simulink model "CMOS_Kernel_Memory_Sync"  (R2023b)
settings: Solver=VariableStepAuto  StartTime=0.0  StopTime=30000000  RelTol=1e-3
values from neighbouring files (symbols this model uses):
  AmountOfPixelsPerScanline = 400    [Kernel_Setup_Script.m]
  AmountOfRamBlocksScanlines = 5    [Kernel_Setup_Script.m]
  AmountOfRamBlocksScanlinesOffset = AmountOfRamBlocksScanlines - 1    (= 4)    [Kernel_Setup_Script.m]
  AmountOfScanlinePixels = 73700    [Kernel_Setup_Script.m]
  AmountOfScanlinePixelsOffset = AmountOfScanlinePixels - 1    (= 73699)    [Kernel_Setup_Script.m]
  AmountOfScanlines = 1100    [Kernel_Setup_Script.m]
  AmountOfScanlinesOffset = AmountOfScanlines - 1    (= 1099)    [Kernel_Setup_Script.m]
  AOPPK_Off = AmountOfPixelsPerScanline - 1    (= 399)    [Kernel_Setup_Script.m]
  AOPPS_Off = AmountOfPixelsPerScanline - 1    (= 399)    [Kernel_Setup_Script.m]
  FramePackOff_0 = FramePackOff_0 - ScanlineFifoCheck    [Kernel_Setup_Script.m]
  FramePackOff_1 = FramePackOff_1 - ScanlineFifoCheck    [Kernel_Setup_Script.m]
  FramePackOff_2 = FramePackOff_2 - ScanlineFifoCheck    [Kernel_Setup_Script.m]
  FramePackOff_3 = FramePackOff_3 - ScanlineFifoCheck    [Kernel_Setup_Script.m]
  FramePackOff_4 = FramePackOff_4 - ScanlineFifoCheck    [Kernel_Setup_Script.m]
  FramePackOff_5 = FramePackOff_5 - ScanlineFifoCheck    [Kernel_Setup_Script.m]
  KernelPackOff_0 = KernelPackOff_0 - KernelBitsPerRow    [Kernel_Setup_Script.m]
  KernelPackOff_1 = KernelPackOff_1 - KernelBitsPerRow    [Kernel_Setup_Script.m]
  KernelPackOff_2 = KernelPackOff_2 - KernelBitsPerRow    [Kernel_Setup_Script.m]
  KernelPackOff_3 = KernelPackOff_3 - KernelBitsPerRow    [Kernel_Setup_Script.m]
  Slice59DownTo48Top = (MsbOffset - (ScanlinePixelBitSizeController*1))    (= 59)    [Kernel_Setup_Script.m]
  Slice71DownTo60Top = (MsbOffset - (ScanlinePixelBitSizeController*0))    (= 71)    [Kernel_Setup_Script.m]
  TotalSectionsForFrames = AmountOfScanlines/AmountOfRamBlocksScanlines    (= 220)    [Kernel_Setup_Script.m]
  UltraRamRows = AmountOfPixelsPerScanline/ScanlineFifoCheck    [Kernel_Setup_Script.m]
  UltraRamRowsCeil = ceil(AmountOfPixelsPerScanline/ScanlineFifoCheck)    [Kernel_Setup_Script.m]
  UltraRamRowsKernel = AmountOfPixelsPerScanline/KernelBitsPerRow    (= 100)    [Kernel_Setup_Script.m]
  UltraRamRowsKernelCeil = ceil(AmountOfPixelsPerScanline/KernelBitsPerRow)    [Kernel_Setup_Script.m]
  UltraRamRowsMemorySectionOffset = UltraRamRowsCeil*AmountOfRamBlocksScanlines    [Kernel_Setup_Script.m]
  UltraRamRowsOffset = UltraRamRowsCeil - 1    [Kernel_Setup_Script.m]
undefined symbols (not defined in the file or in its folder): c, Down, sfvc784, Up, xck26
libraries: hdlBasic x4512, vmcUtilities x1
(part 14 of 39)

== system CMOS_Kernel_Memory_Sync/Memory Handler/Data Slicer/Frame RAM Slicer/72 Bit Unpacker RAM 4 ==
  Data In : Inport
  Enable : Inport  Port=2
  Read Enable : Inport  Port=3
  Last Point : Inport  Port=4
  72bit Frame FIFO 0 : hdlBasic/FIFO  mem_type=Block RAM  performance_options=Standard_FIFO  embedded_registers=off  depth=16  use_asym_data_widths=off  asym_read_width=32  percent_nbits=1  rst=off  rst_latency=2  en=off  use_dcount=off  use_percent_full_port=off  use_almost_empty=off  almost_empty_thresh=2  use_almost_full=off  use_rd_rst_busy=off  use_wr_rst_busy=off  almost_full_thresh=14  almost_empty_offset=[]  almost_full_offset=[]  explicit_period=off  period=[]  store_only_valid=[]  init_zero=[]  simulation_type=fast_sim  XmcBlockStatus=1  maskContainerNames=tabcontainer1  block_type=fifo  block_config=sysgen:FIFO_config  block_width=538  block_height=997
      settings: infoedit=[]
  72bit Frame FIFO 1 : hdlBasic/FIFO  mem_type=Block RAM  performance_options=Standard_FIFO  embedded_registers=off  depth=16  use_asym_data_widths=off  asym_read_width=32  percent_nbits=1  rst=off  rst_latency=2  en=off  use_dcount=off  use_percent_full_port=off  use_almost_empty=off  almost_empty_thresh=2  use_almost_full=off  use_rd_rst_busy=off  use_wr_rst_busy=off  almost_full_thresh=14  almost_empty_offset=[]  almost_full_offset=[]  explicit_period=off  period=[]  store_only_valid=[]  init_zero=[]  simulation_type=fast_sim  XmcBlockStatus=1  maskContainerNames=tabcontainer1  block_type=fifo  block_config=sysgen:FIFO_config  block_width=538  block_height=997
      settings: infoedit=[]
  Bypass Delay : hdlBasic/Delay  rst=off  en=off  latency=1  reg_retiming=off  XmcBlockStatus=1  maskContainerNames=group1  block_type=delay  block_config=sysgen:Delay_config
  Bypass Delay1 : hdlBasic/Delay  rst=off  en=off  latency=1  reg_retiming=off  XmcBlockStatus=1  maskContainerNames=group1  block_type=delay  block_config=sysgen:Delay_config
  Bypass Delay2 : hdlBasic/Delay  rst=off  en=off  latency=1  reg_retiming=off  XmcBlockStatus=1  maskContainerNames=group1  block_type=delay  block_config=sysgen:Delay_config
  Data Delay : hdlBasic/Delay  rst=off  en=off  latency=1  reg_retiming=off  XmcBlockStatus=1  maskContainerNames=group1  block_type=delay  block_config=sysgen:Delay_config
  Data Enable Check : hdlBasic/Delay  rst=off  en=off  latency=1  reg_retiming=off  XmcBlockStatus=1  maskContainerNames=group1  block_type=delay  block_config=sysgen:Delay_config
  Data MUX Delay : hdlBasic/Delay  rst=off  en=off  latency=1  reg_retiming=off  XmcBlockStatus=1  maskContainerNames=group1  block_type=delay  block_config=sysgen:Delay_config
  Enable Delay : hdlBasic/Delay  rst=off  en=off  latency=1  reg_retiming=off  XmcBlockStatus=1  maskContainerNames=group1  block_type=delay  block_config=sysgen:Delay_config
  FIFO 0 : hdlBasic/Constant  const=0  gui_display_data_type=Fixed-point  arith_type=Unsigned  n_bits=1  bin_pt=0  preci_type=Single  exp_width=8  frac_width=24  explicit_period=off  period=1  XmcBlockStatus=1  maskContainerNames=tabcontainer1  block_type=constant  block_config=sysgen:Constant_config
  FIFO 1 : hdlBasic/Constant  const=1  gui_display_data_type=Fixed-point  arith_type=Unsigned  n_bits=1  bin_pt=0  preci_type=Single  exp_width=8  frac_width=24  explicit_period=off  period=1  XmcBlockStatus=1  maskContainerNames=tabcontainer1  block_type=constant  block_config=sysgen:Constant_config
  Last Point Delay 1 : hdlBasic/Delay  rst=off  en=off  latency=1  reg_retiming=off  XmcBlockStatus=1  maskContainerNames=group1  block_type=delay  block_config=sysgen:Delay_config
  Last Value Bypass FIFO 0 : hdlBasic/Logical  logical_function=OR  inputs=2  en=off  latency=1  precision=Full  arith_type=Unsigned  n_bits=16  bin_pt=0  align_bp=on  overflow=[]  quantization=[]  XmcBlockStatus=1  maskContainerNames=tabcontainer1  block_type=logical  block_config=sysgen:Logical_config
  Last Value Bypass FIFO 1 : hdlBasic/Logical  logical_function=OR  inputs=2  en=off  latency=1  precision=Full  arith_type=Unsigned  n_bits=16  bin_pt=0  align_bp=on  overflow=[]  quantization=[]  XmcBlockStatus=1  maskContainerNames=tabcontainer1  block_type=logical  block_config=sysgen:Logical_config
  Last Value Delay : hdlBasic/Delay  rst=off  en=off  latency=1  reg_retiming=off  XmcBlockStatus=1  maskContainerNames=group1  block_type=delay  block_config=sysgen:Delay_config
  Logical : hdlBasic/Logical  logical_function=NOR  inputs=2  en=off  latency=1  precision=Full  arith_type=Unsigned  n_bits=16  bin_pt=0  align_bp=on  overflow=[]  quantization=[]  XmcBlockStatus=1  maskContainerNames=tabcontainer1  block_type=logical  block_config=sysgen:Logical_config
  Store in FIFO 0 : hdlBasic/Relational  mode=a=b  op_type=Bool  en=off  latency=1  XmcBlockStatus=1  maskContainerNames=tabcontainer1  block_type=relational  block_config=sysgen:Relational_config
  Store in FIFO 1 : hdlBasic/Relational  mode=a=b  op_type=Bool  en=off  latency=1  XmcBlockStatus=1  maskContainerNames=tabcontainer1  block_type=relational  block_config=sysgen:Relational_config
  Sync Frame Counter : hdlBasic/Counter  cnt_type=Count limited  cnt_to=1  operation=Up  start_count=0  cnt_by_val=1  arith_type=Unsigned  n_bits=1  bin_pt=0  load_pin=off  rst=on  en=on  explicit_period=Explicit  period=1  use_behavioral_HDL=off  implementation=Fabric  XmcBlockStatus=1  maskContainerNames=group1  block_type=counter  block_config=sysgen:Counter_config  block_width=531  block_height=1023
  Unpack 72 Bit FIFO 0 : Subsystem
      settings: RTWMemSecFuncInitTerm=Inherit fRAM model  RTWMemSecFuncExecute=Inherit fRAM model  RTWMemSecDataConstants=Inherit fRAM model  RTWMemSecDataInternal=Inherit fRAM model  RTWMemSecDataParameters=Inherit fRAM model
  Unpack 72 Bit FIFO 1 : Subsystem
      settings: RTWMemSecFuncInitTerm=Inherit fRAM model  RTWMemSecFuncExecute=Inherit fRAM model  RTWMemSecDataConstants=Inherit fRAM model  RTWMemSecDataInternal=Inherit fRAM model  RTWMemSecDataParameters=Inherit fRAM model
  Valid : hdlBasic/Delay  rst=off  en=off  latency=1  reg_retiming=off  XmcBlockStatus=1  maskContainerNames=group1  block_type=delay  block_config=sysgen:Delay_config
  Write FIFO 0 MUX Delay : hdlBasic/Delay  rst=off  en=off  latency=1  reg_retiming=off  XmcBlockStatus=1  maskContainerNames=group1  block_type=delay  block_config=sysgen:Delay_config
  Write FIFO 1 MUX Delay : hdlBasic/Delay  rst=off  en=off  latency=1  reg_retiming=off  XmcBlockStatus=1  maskContainerNames=group1  block_type=delay  block_config=sysgen:Delay_config
  Write to FIFO 0 : hdlBasic/Logical  logical_function=AND  inputs=2  en=off  latency=1  precision=Full  arith_type=Unsigned  n_bits=16  bin_pt=0  align_bp=on  overflow=[]  quantization=[]  XmcBlockStatus=1  maskContainerNames=tabcontainer1  block_type=logical  block_config=sysgen:Logical_config
  Write to FIFO 1 : hdlBasic/Logical  logical_function=AND  inputs=2  en=off  latency=1  precision=Full  arith_type=Unsigned  n_bits=16  bin_pt=0  align_bp=on  overflow=[]  quantization=[]  XmcBlockStatus=1  maskContainerNames=tabcontainer1  block_type=logical  block_config=sysgen:Logical_config
  Zero FIFO Value : hdlBasic/Constant  const=0  gui_display_data_type=Fixed-point  arith_type=Unsigned  n_bits=72  bin_pt=0  preci_type=Single  exp_width=8  frac_width=24  explicit_period=off  period=1  XmcBlockStatus=1  maskContainerNames=tabcontainer1  block_type=constant  block_config=sysgen:Constant_config
  Zero Value : hdlBasic/Mux  inputs=2  en=off  latency=1  precision=Full  arith_type=Unsigned  n_bits=16  bin_pt=14  quantization=Truncate  overflow=Wrap  XmcBlockStatus=1  maskContainerNames=tabcontainer1  block_type=mux  block_config=sysgen:Mux_config
  71 Downto 60 FIFO 0 : Outport
  59 Downto 48 FIFO 0 : Outport  Port=2
  47 Downto 36 FIFO 0 : Outport  Port=3
  35 Downto 24 FIFO 0 : Outport  Port=4
  23 Downto 12 FIFO 0 : Outport  Port=5
  11 Downto 0 FIFO 0 : Outport  Port=6
  71 Downto 60 FIFO 1 : Outport  Port=7
  59 Downto 48 FIFO 1 : Outport  Port=8
  47 Downto 36 FIFO 1 : Outport  Port=9
  35 Downto 24 FIFO 1 : Outport  Port=10
  23 Downto 12 FIFO 1 : Outport  Port=11
  11 Downto 0 FIFO 1 : Outport  Port=12
  Valid Out : Outport  Port=13
  Wrote To a FIFO : Outport  Port=14
  wires:
  Sync Frame Counter/1 -> Store in FIFO 1/1, Store in FIFO 0/1
  Read Enable/1 -> 72bit Frame FIFO 0/3, 72bit Frame FIFO 1/3, Valid/1
  FIFO 1/1 -> Store in FIFO 1/2
  FIFO 0/1 -> Store in FIFO 0/2
  Write to FIFO 1/1 -> Write FIFO 1 MUX Delay/1
  Data Delay/1 -> Data Enable Check/1
  Data In/1 -> Data Delay/1
  Enable/1 -> Enable Delay/1, Sync Frame Counter/2
  72bit Frame FIFO 1/1 -> Unpack 72 Bit FIFO 1/1(72 Bit Input)
  72bit Frame FIFO 0/1 -> Unpack 72 Bit FIFO 0/1(72 Bit Input)
  Unpack 72 Bit FIFO 0/1(71 Downto 60) -> 71 Downto 60 FIFO 0/1
  Unpack 72 Bit FIFO 0/2(59 Downto 48) -> 59 Downto 48 FIFO 0/1
  Unpack 72 Bit FIFO 0/3(47 Downto 36) -> 47 Downto 36 FIFO 0/1
  Unpack 72 Bit FIFO 0/4(35 Downto 24) -> 35 Downto 24 FIFO 0/1
  Unpack 72 Bit FIFO 0/5(23 Downto 12) -> 23 Downto 12 FIFO 0/1
  Unpack 72 Bit FIFO 0/6(11 Downto 0) -> 11 Downto 0 FIFO 0/1
  Unpack 72 Bit FIFO 1/1(71 Downto 60) -> 71 Downto 60 FIFO 1/1
  Unpack 72 Bit FIFO 1/2(59 Downto 48) -> 59 Downto 48 FIFO 1/1
  Unpack 72 Bit FIFO 1/3(47 Downto 36) -> 47 Downto 36 FIFO 1/1
  Unpack 72 Bit FIFO 1/4(35 Downto 24) -> 35 Downto 24 FIFO 1/1
  Unpack 72 Bit FIFO 1/5(23 Downto 12) -> 23 Downto 12 FIFO 1/1
  Unpack 72 Bit FIFO 1/6(11 Downto 0) -> 11 Downto 0 FIFO 1/1
  Valid/1 -> Valid Out/1
  Write to FIFO 0/1 -> Write FIFO 0 MUX Delay/1
  Data Enable Check/1 -> Last Value Delay/1
  Enable Delay/1 -> Bypass Delay/1
  Last Point/1 -> Last Point Delay 1/1, Sync Frame Counter/1
  Last Value Delay/1 -> Data MUX Delay/1, Zero Value/2
  Last Value Bypass FIFO 0/1 -> Write to FIFO 0/1
  Store in FIFO 0/1 -> Last Value Bypass FIFO 0/1
  Last Value Bypass FIFO 1/1 -> Write to FIFO 1/2
  Store in FIFO 1/1 -> Last Value Bypass FIFO 1/1
  Last Point Delay 1/1 -> Last Value Bypass FIFO 1/2, Last Value Bypass FIFO 0/2, Bypass Delay1/1
  Bypass Delay/1 -> Write to FIFO 1/1, Write to FIFO 0/2
  Logical/1 -> Wrote To a FIFO/1
  72bit Frame FIFO 1/2 -> Logical/2
  72bit Frame FIFO 0/2 -> Logical/1
  Zero FIFO Value/1 -> Zero Value/3
  Zero Value/1 -> 72bit Frame FIFO 1/1
  Write FIFO 1 MUX Delay/1 -> 72bit Frame FIFO 1/2
  Write FIFO 0 MUX Delay/1 -> 72bit Frame FIFO 0/2
  Data MUX Delay/1 -> 72bit Frame FIFO 0/1
  Bypass Delay1/1 -> Bypass Delay2/1
  Bypass Delay2/1 -> Zero Value/1

== system CMOS_Kernel_Memory_Sync/Memory Handler/Data Slicer/Frame RAM Slicer/Data Point Tracker ==
  Data In RAM 0 : Inport
  Data In RAM 1 : Inport  Port=2
  Data In RAM 2 : Inport  Port=3
  Data In RAM 3 : Inport  Port=4
  Data In RAM 4 : Inport  Port=5
  Valid Enable In : Inport  Port=6
  Data In Delay 0 RAM {0..4} (5 alike) : hdlBasic/Delay  rst=off  en=off  latency=1  reg_retiming=off  XmcBlockStatus=1  maskContainerNames=group1  block_type=delay  block_config=sysgen:Delay_config
  Data In Delay 1 RAM {0..4} (5 alike) : hdlBasic/Delay  rst=off  en=off  latency=1  reg_retiming=off  XmcBlockStatus=1  maskContainerNames=group1  block_type=delay  block_config=sysgen:Delay_config
  Data Point Counter : hdlBasic/Counter  cnt_type=Count limited  cnt_to=UltraRamRowsCeil - 1  operation=Up  start_count=0  cnt_by_val=1  arith_type=Unsigned  n_bits=ceil(log2(UltraRamRowsCeil))  bin_pt=0  load_pin=off  rst=off  en=on  explicit_period=Explicit  period=1  use_behavioral_HDL=off  implementation=Fabric  XmcBlockStatus=1  maskContainerNames=group1  block_type=counter  block_config=sysgen:Counter_config  block_width=531  block_height=1023
  Last Data Point Value : hdlBasic/Constant  const=UltraRamRowsCeil - 1  gui_display_data_type=Fixed-point  arith_type=Unsigned  n_bits=ceil(log2(UltraRamRowsCeil))  bin_pt=0  preci_type=Single  exp_width=8  frac_width=24  explicit_period=off  period=1  XmcBlockStatus=1  maskContainerNames=tabcontainer1  block_type=constant  block_config=sysgen:Constant_config
  Last Point : hdlBasic/Relational  mode=a=b  op_type=Bool  en=off  latency=1  XmcBlockStatus=1  maskContainerNames=tabcontainer1  block_type=relational  block_config=sysgen:Relational_config
  Last Value enable : hdlBasic/Logical  logical_function=AND  inputs=2  en=off  latency=1  precision=Full  arith_type=Unsigned  n_bits=16  bin_pt=0  align_bp=on  overflow=[]  quantization=[]  XmcBlockStatus=1  maskContainerNames=tabcontainer1  block_type=logical  block_config=sysgen:Logical_config
  Valid Delay 0 : hdlBasic/Delay  rst=off  en=off  latency=1  reg_retiming=off  XmcBlockStatus=1  maskContainerNames=group1  block_type=delay  block_config=sysgen:Delay_config
  Valid Delay 1 : hdlBasic/Delay  rst=off  en=off  latency=1  reg_retiming=off  XmcBlockStatus=1  maskContainerNames=group1  block_type=delay  block_config=sysgen:Delay_config
  Data Out RAM 0 : Outport
  Data Out RAM 1 : Outport  Port=2
  Data Out RAM 2 : Outport  Port=3
  Data Out RAM 3 : Outport  Port=4
  Data Out RAM 4 : Outport  Port=5
  Valid Enable Out : Outport  Port=6
  Last Value Out : Outport  Port=7
  wires:
  Last Value enable/1 -> Last Value Out/1
  Data In Delay 0 RAM 1/1 -> Data In Delay 1 RAM 1/1
  Last Point/1 -> Last Value enable/2
  Data Point Counter/1 -> Last Point/1
  Valid Enable In/1 -> Valid Delay 0/1, Data Point Counter/1
  Data In Delay 0 RAM 2/1 -> Data In Delay 1 RAM 2/1
  Valid Delay 0/1 -> Last Value enable/1, Valid Delay 1/1
  Last Data Point Value/1 -> Last Point/2
  Data In Delay 0 RAM 4/1 -> Data In Delay 1 RAM 4/1
  Data In Delay 1 RAM 4/1 -> Data Out RAM 4/1
  Data In Delay 0 RAM 0/1 -> Data In Delay 1 RAM 0/1
  Data In Delay 0 RAM 3/1 -> Data In Delay 1 RAM 3/1
  Data In RAM 1/1 -> Data In Delay 0 RAM 1/1
  Data In Delay 1 RAM 0/1 -> Data Out RAM 0/1
  Data In RAM 3/1 -> Data In Delay 0 RAM 3/1
  Data In RAM 4/1 -> Data In Delay 0 RAM 4/1
  Data In RAM 2/1 -> Data In Delay 0 RAM 2/1
  Data In RAM 0/1 -> Data In Delay 0 RAM 0/1
  Data In Delay 1 RAM 2/1 -> Data Out RAM 2/1
  Data In Delay 1 RAM 3/1 -> Data Out RAM 3/1
  Data In Delay 1 RAM 1/1 -> Data Out RAM 1/1
  Valid Delay 1/1 -> Valid Enable Out/1

== system CMOS_Kernel_Memory_Sync/Memory Handler/Data Slicer/Kernel RAM Slicer/72 Bit Kernel Unpacker RAM 0 ==
  Data In : Inport
  Enable : Inport  Port=2
  Read Enable : Inport  Port=3
  Last Point : Inport  Port=4
  72bit Frame FIFO 0 : hdlBasic/FIFO  mem_type=Block RAM  performance_options=Standard_FIFO  embedded_registers=off  depth=16  use_asym_data_widths=off  asym_read_width=32  percent_nbits=1  rst=off  rst_latency=2  en=off  use_dcount=off  use_percent_full_port=off  use_almost_empty=off  almost_empty_thresh=2  use_almost_full=off  use_rd_rst_busy=off  use_wr_rst_busy=off  almost_full_thresh=14  almost_empty_offset=[]  almost_full_offset=[]  explicit_period=off  period=[]  store_only_valid=[]  init_zero=[]  simulation_type=fast_sim  XmcBlockStatus=1  maskContainerNames=tabcontainer1  block_type=fifo  block_config=sysgen:FIFO_config  block_width=538  block_height=997
      settings: infoedit=[]
  72bit Frame FIFO 1 : hdlBasic/FIFO  mem_type=Block RAM  performance_options=Standard_FIFO  embedded_registers=off  depth=16  use_asym_data_widths=off  asym_read_width=32  percent_nbits=1  rst=off  rst_latency=2  en=off  use_dcount=off  use_percent_full_port=off  use_almost_empty=off  almost_empty_thresh=2  use_almost_full=off  use_rd_rst_busy=off  use_wr_rst_busy=off  almost_full_thresh=14  almost_empty_offset=[]  almost_full_offset=[]  explicit_period=off  period=[]  store_only_valid=[]  init_zero=[]  simulation_type=fast_sim  XmcBlockStatus=1  maskContainerNames=tabcontainer1  block_type=fifo  block_config=sysgen:FIFO_config  block_width=538  block_height=997
      settings: infoedit=[]
  72bit Frame FIFO 2 : hdlBasic/FIFO  mem_type=Block RAM  performance_options=Standard_FIFO  embedded_registers=off  depth=16  use_asym_data_widths=off  asym_read_width=32  percent_nbits=1  rst=off  rst_latency=2  en=off  use_dcount=off  use_percent_full_port=off  use_almost_empty=off  almost_empty_thresh=2  use_almost_full=off  use_rd_rst_busy=off  use_wr_rst_busy=off  almost_full_thresh=14  almost_empty_offset=[]  almost_full_offset=[]  explicit_period=off  period=[]  store_only_valid=[]  init_zero=[]  simulation_type=fast_sim  XmcBlockStatus=1  maskContainerNames=tabcontainer1  block_type=fifo  block_config=sysgen:FIFO_config  block_width=538  block_height=997
      settings: infoedit=[]
  Bypass Delay : hdlBasic/Delay  rst=off  en=off  latency=1  reg_retiming=off  XmcBlockStatus=1  maskContainerNames=group1  block_type=delay  block_config=sysgen:Delay_config
  Data Delay {0..8} (9 alike) : hdlBasic/Delay  rst=off  en=off  latency=1  reg_retiming=off  XmcBlockStatus=1  maskContainerNames=group1  block_type=delay  block_config=sysgen:Delay_config
  Enable Delay : hdlBasic/Delay  rst=off  en=off  latency=1  reg_retiming=off  XmcBlockStatus=1  maskContainerNames=group1  block_type=delay  block_config=sysgen:Delay_config
  FIFO 0 : hdlBasic/Constant  const=0  gui_display_data_type=Fixed-point  arith_type=Unsigned  n_bits=1  bin_pt=0  preci_type=Single  exp_width=8  frac_width=24  explicit_period=off  period=1  XmcBlockStatus=1  maskContainerNames=tabcontainer1  block_type=constant  block_config=sysgen:Constant_config
  FIFO 1 : hdlBasic/Constant  const=1  gui_display_data_type=Fixed-point  arith_type=Unsigned  n_bits=1  bin_pt=0  preci_type=Single  exp_width=8  frac_width=24  explicit_period=off  period=1  XmcBlockStatus=1  maskContainerNames=tabcontainer1  block_type=constant  block_config=sysgen:Constant_config
  FIFO 2 : hdlBasic/Constant  const=2  gui_display_data_type=Fixed-point  arith_type=Unsigned  n_bits=2  bin_pt=0  preci_type=Single  exp_width=8  frac_width=24  explicit_period=off  period=1  XmcBlockStatus=1  maskContainerNames=tabcontainer1  block_type=constant  block_config=sysgen:Constant_config
  "Last FIFO Written to " : hdlBasic/Delay  rst=off  en=off  latency=1  reg_retiming=off  XmcBlockStatus=1  maskContainerNames=group1  block_type=delay  block_config=sysgen:Delay_config
  Last FIFO Written to 1 : hdlBasic/Delay  rst=off  en=off  latency=1  reg_retiming=off  XmcBlockStatus=1  maskContainerNames=group1  block_type=delay  block_config=sysgen:Delay_config
  Last Point Delay : hdlBasic/Delay  rst=off  en=off  latency=1  reg_retiming=off  XmcBlockStatus=1  maskContainerNames=group1  block_type=delay  block_config=sysgen:Delay_config
  Last Value Bypass FIFO 0 : hdlBasic/Logical  logical_function=OR  inputs=2  en=off  latency=1  precision=Full  arith_type=Unsigned  n_bits=16  bin_pt=0  align_bp=on  overflow=[]  quantization=[]  XmcBlockStatus=1  maskContainerNames=tabcontainer1  block_type=logical  block_config=sysgen:Logical_config
  Last Value Bypass FIFO 1 : hdlBasic/Logical  logical_function=OR  inputs=2  en=off  latency=1  precision=Full  arith_type=Unsigned  n_bits=16  bin_pt=0  align_bp=on  overflow=[]  quantization=[]  XmcBlockStatus=1  maskContainerNames=tabcontainer1  block_type=logical  block_config=sysgen:Logical_config
  Last Value Bypass FIFO 2 : hdlBasic/Logical  logical_function=OR  inputs=2  en=off  latency=1  precision=Full  arith_type=Unsigned  n_bits=16  bin_pt=0  align_bp=on  overflow=[]  quantization=[]  XmcBlockStatus=1  maskContainerNames=tabcontainer1  block_type=logical  block_config=sysgen:Logical_config
  Logical : hdlBasic/Logical  logical_function=NOR  inputs=3  en=off  latency=1  precision=Full  arith_type=Unsigned  n_bits=16  bin_pt=0  align_bp=on  overflow=[]  quantization=[]  XmcBlockStatus=1  maskContainerNames=tabcontainer1  block_type=logical  block_config=sysgen:Logical_config
  Store in FIFO 0 : hdlBasic/Relational  mode=a=b  op_type=Bool  en=off  latency=1  XmcBlockStatus=1  maskContainerNames=tabcontainer1  block_type=relational  block_config=sysgen:Relational_config
  Store in FIFO 1 : hdlBasic/Relational  mode=a=b  op_type=Bool  en=off  latency=1  XmcBlockStatus=1  maskContainerNames=tabcontainer1  block_type=relational  block_config=sysgen:Relational_config
  Store in FIFO 2 : hdlBasic/Relational  mode=a=b  op_type=Bool  en=off  latency=1  XmcBlockStatus=1  maskContainerNames=tabcontainer1  block_type=relational  block_config=sysgen:Relational_config
  Sync Frame Counter : hdlBasic/Counter  cnt_type=Count limited  cnt_to=2  operation=Up  start_count=0  cnt_by_val=1  arith_type=Unsigned  n_bits=2  bin_pt=0  load_pin=off  rst=on  en=on  explicit_period=Explicit  period=1  use_behavioral_HDL=off  implementation=Fabric  XmcBlockStatus=1  maskContainerNames=group1  block_type=counter  block_config=sysgen:Counter_config  block_width=531  block_height=1023
  Unpack Kernel 72 Bit FIFO 0 : Subsystem
      settings: RTWMemSecFuncInitTerm=Inherit fRAM model  RTWMemSecFuncExecute=Inherit fRAM model  RTWMemSecDataConstants=Inherit fRAM model  RTWMemSecDataInternal=Inherit fRAM model  RTWMemSecDataParameters=Inherit fRAM model
  Unpack Kernel 72 Bit FIFO 1 : Subsystem
      settings: RTWMemSecFuncInitTerm=Inherit fRAM model  RTWMemSecFuncExecute=Inherit fRAM model  RTWMemSecDataConstants=Inherit fRAM model  RTWMemSecDataInternal=Inherit fRAM model  RTWMemSecDataParameters=Inherit fRAM model
  Unpack Kernel 72 Bit FIFO 2 : Subsystem
      settings: RTWMemSecFuncInitTerm=Inherit fRAM model  RTWMemSecFuncExecute=Inherit fRAM model  RTWMemSecDataConstants=Inherit fRAM model  RTWMemSecDataInternal=Inherit fRAM model  RTWMemSecDataParameters=Inherit fRAM model
  Valid : hdlBasic/Delay  rst=off  en=off  latency=1  reg_retiming=off  XmcBlockStatus=1  maskContainerNames=group1  block_type=delay  block_config=sysgen:Delay_config
  Write to FIFO 0 : hdlBasic/Logical  logical_function=AND  inputs=2  en=off  latency=1  precision=Full  arith_type=Unsigned  n_bits=16  bin_pt=0  align_bp=on  overflow=[]  quantization=[]  XmcBlockStatus=1  maskContainerNames=tabcontainer1  block_type=logical  block_config=sysgen:Logical_config
  Write to FIFO 1 : hdlBasic/Logical  logical_function=AND  inputs=2  en=off  latency=1  precision=Full  arith_type=Unsigned  n_bits=16  bin_pt=0  align_bp=on  overflow=[]  quantization=[]  XmcBlockStatus=1  maskContainerNames=tabcontainer1  block_type=logical  block_config=sysgen:Logical_config
  Write to FIFO 2 : hdlBasic/Logical  logical_function=AND  inputs=2  en=off  latency=1  precision=Full  arith_type=Unsigned  n_bits=16  bin_pt=0  align_bp=on  overflow=[]  quantization=[]  XmcBlockStatus=1  maskContainerNames=tabcontainer1  block_type=logical  block_config=sysgen:Logical_config
  Zero Out : hdlBasic/Constant  const=0  gui_display_data_type=Fixed-point  arith_type=Unsigned  n_bits=72  bin_pt=0  preci_type=Single  exp_width=8  frac_width=24  explicit_period=off  period=1  XmcBlockStatus=1  maskContainerNames=tabcontainer1  block_type=constant  block_config=sysgen:Constant_config
  Zero Value : hdlBasic/Mux  inputs=2  en=off  latency=1  precision=Full  arith_type=Unsigned  n_bits=16  bin_pt=14  quantization=Truncate  overflow=Wrap  XmcBlockStatus=1  maskContainerNames=tabcontainer1  block_type=mux  block_config=sysgen:Mux_config
  71 Downto 54 FIFO 0 : Outport
  53 Downto 36 FIFO 0 : Outport  Port=2
  35 Downto 18 FIFO 0 : Outport  Port=3
  17 Downto 0 FIFO 0 : Outport  Port=4
  71 Downto 54 FIFO 1 : Outport  Port=5
  53 Downto 36 FIFO 1 : Outport  Port=6
  35 Downto 18 FIFO 1 : Outport  Port=7
  17 Downto 0 FIFO 1 : Outport  Port=8
  71 Downto 54 FIFO 2 : Outport  Port=9
  53 Downto 36 FIFO 2 : Outport  Port=10
  35 Downto 18 FIFO 2 : Outport  Port=11
  17 Downto 0 FIFO 2 : Outport  Port=12
  Valid Out : Outport  Port=13
  Wrote To a FIFO : Outport  Port=14
  Wrote to last FIFO : Outport  Port=15
  wires:
  Sync Frame Counter/1 -> Store in FIFO 2/1, Store in FIFO 1/1, Store in FIFO 0/1
  FIFO 1/1 -> Store in FIFO 1/2
  FIFO 0/1 -> Store in FIFO 0/2
  Data Delay 0/1 -> Data Delay 1/1
  Data In/1 -> Data Delay 0/1
  Enable/1 -> Enable Delay/1, Sync Frame Counter/2
  72bit Frame FIFO 0/1 -> Unpack Kernel 72 Bit FIFO 0/1(72 Bit Input)
  Unpack Kernel 72 Bit FIFO 0/1(71 Downto 54) -> 71 Downto 54 FIFO 0/1
  Unpack Kernel 72 Bit FIFO 0/2(53 Downto 36) -> 53 Downto 36 FIFO 0/1
  Unpack Kernel 72 Bit FIFO 0/3(35 Downto 18) -> 35 Downto 18 FIFO 0/1
  Unpack Kernel 72 Bit FIFO 0/4(17 Downto 0) -> 17 Downto 0 FIFO 0/1
  Valid/1 -> Valid Out/1
  FIFO 2/1 -> Store in FIFO 2/2
  Unpack Kernel 72 Bit FIFO 1/3(35 Downto 18) -> 35 Downto 18 FIFO 1/1
  Unpack Kernel 72 Bit FIFO 1/2(53 Downto 36) -> 53 Downto 36 FIFO 1/1
  Unpack Kernel 72 Bit FIFO 1/1(71 Downto 54) -> 71 Downto 54 FIFO 1/1
  Unpack Kernel 72 Bit FIFO 1/4(17 Downto 0) -> 17 Downto 0 FIFO 1/1
  72bit Frame FIFO 1/1 -> Unpack Kernel 72 Bit FIFO 1/1(72 Bit Input)
  Unpack Kernel 72 Bit FIFO 2/3(35 Downto 18) -> 35 Downto 18 FIFO 2/1
  Unpack Kernel 72 Bit FIFO 2/2(53 Downto 36) -> 53 Downto 36 FIFO 2/1
  Unpack Kernel 72 Bit FIFO 2/1(71 Downto 54) -> 71 Downto 54 FIFO 2/1
  Unpack Kernel 72 Bit FIFO 2/4(17 Downto 0) -> 17 Downto 0 FIFO 2/1
  72bit Frame FIFO 2/1 -> Unpack Kernel 72 Bit FIFO 2/1(72 Bit Input)
  Last Value Bypass FIFO 0/1 -> Write to FIFO 0/1
  Last Value Bypass FIFO 1/1 -> Write to FIFO 1/2
  Bypass Delay/1 -> Write to FIFO 1/1, Write to FIFO 2/1, Write to FIFO 0/2
  Last Value Bypass FIFO 2/1 -> Write to FIFO 2/2
  Write to FIFO 0/1 -> Data Delay 4/1
  Write to FIFO 1/1 -> Data Delay 5/1
  Write to FIFO 2/1 -> Data Delay 6/1
  Store in FIFO 0/1 -> Last Value Bypass FIFO 0/2
  Store in FIFO 1/1 -> Last Value Bypass FIFO 1/1
  Store in FIFO 2/1 -> Last Value Bypass FIFO 2/1
  Enable Delay/1 -> Bypass Delay/1
  Last Point/1 -> Last Point Delay/1, Sync Frame Counter/1
  Last Point Delay/1 -> Last Value Bypass FIFO 2/2, Last Value Bypass FIFO 0/1, Data Delay 7/1, Last Value Bypass FIFO 1/2
  Data Delay 1/1 -> Data Delay 2/1
  Data Delay 2/1 -> Data Delay 3/1, Zero Value/2
  Logical/1 -> Wrote To a FIFO/1
  72bit Frame FIFO 1/2 -> Logical/1
  72bit Frame FIFO 2/2 -> Logical/2
  72bit Frame FIFO 0/2 -> Logical/3
  Read Enable/1 -> 72bit Frame FIFO 0/3, 72bit Frame FIFO 1/3, 72bit Frame FIFO 2/3, Valid/1
  "Last FIFO Written to "/1 -> Last FIFO Written to 1/1
  Last FIFO Written to 1/1 -> Wrote to last FIFO/1
  Data Delay 5/1 -> 72bit Frame FIFO 1/2
  Data Delay 6/1 -> 72bit Frame FIFO 2/2, "Last FIFO Written to "/1
  Data Delay 3/1 -> 72bit Frame FIFO 0/1
  Data Delay 4/1 -> 72bit Frame FIFO 0/2
  Zero Value/1 -> 72bit Frame FIFO 1/1, 72bit Frame FIFO 2/1
  Data Delay 7/1 -> Data Delay 8/1
  Data Delay 8/1 -> Zero Value/1
  Zero Out/1 -> Zero Value/3

== system CMOS_Kernel_Memory_Sync/Memory Handler/Data Slicer/Kernel RAM Slicer/72 Bit Kernel Unpacker RAM 1 ==
  Data In : Inport
  Enable : Inport  Port=2
  Read Enable : Inport  Port=3
  Last Point : Inport  Port=4
  72bit Frame FIFO 0 : hdlBasic/FIFO  mem_type=Block RAM  performance_options=Standard_FIFO  embedded_registers=off  depth=16  use_asym_data_widths=off  asym_read_width=32  percent_nbits=1  rst=off  rst_latency=2  en=off  use_dcount=off  use_percent_full_port=off  use_almost_empty=off  almost_empty_thresh=2  use_almost_full=off  use_rd_rst_busy=off  use_wr_rst_busy=off  almost_full_thresh=14  almost_empty_offset=[]  almost_full_offset=[]  explicit_period=off  period=[]  store_only_valid=[]  init_zero=[]  simulation_type=fast_sim  XmcBlockStatus=1  maskContainerNames=tabcontainer1  block_type=fifo  block_config=sysgen:FIFO_config  block_width=538  block_height=997
      settings: infoedit=[]
  72bit Frame FIFO 1 : hdlBasic/FIFO  mem_type=Block RAM  performance_options=Standard_FIFO  embedded_registers=off  depth=16  use_asym_data_widths=off  asym_read_width=32  percent_nbits=1  rst=off  rst_latency=2  en=off  use_dcount=off  use_percent_full_port=off  use_almost_empty=off  almost_empty_thresh=2  use_almost_full=off  use_rd_rst_busy=off  use_wr_rst_busy=off  almost_full_thresh=14  almost_empty_offset=[]  almost_full_offset=[]  explicit_period=off  period=[]  store_only_valid=[]  init_zero=[]  simulation_type=fast_sim  XmcBlockStatus=1  maskContainerNames=tabcontainer1  block_type=fifo  block_config=sysgen:FIFO_config  block_width=538  block_height=997
      settings: infoedit=[]
  72bit Frame FIFO 2 : hdlBasic/FIFO  mem_type=Block RAM  performance_options=Standard_FIFO  embedded_registers=off  depth=16  use_asym_data_widths=off  asym_read_width=32  percent_nbits=1  rst=off  rst_latency=2  en=off  use_dcount=off  use_percent_full_port=off  use_almost_empty=off  almost_empty_thresh=2  use_almost_full=off  use_rd_rst_busy=off  use_wr_rst_busy=off  almost_full_thresh=14  almost_empty_offset=[]  almost_full_offset=[]  explicit_period=off  period=[]  store_only_valid=[]  init_zero=[]  simulation_type=fast_sim  XmcBlockStatus=1  maskContainerNames=tabcontainer1  block_type=fifo  block_config=sysgen:FIFO_config  block_width=538  block_height=997
      settings: infoedit=[]
  Bypass Delay : hdlBasic/Delay  rst=off  en=off  latency=1  reg_retiming=off  XmcBlockStatus=1  maskContainerNames=group1  block_type=delay  block_config=sysgen:Delay_config
  Bypass Delay1 : hdlBasic/Delay  rst=off  en=off  latency=1  reg_retiming=off  XmcBlockStatus=1  maskContainerNames=group1  block_type=delay  block_config=sysgen:Delay_config
  Bypass Delay2 : hdlBasic/Delay  rst=off  en=off  latency=1  reg_retiming=off  XmcBlockStatus=1  maskContainerNames=group1  block_type=delay  block_config=sysgen:Delay_config
  Data Delay {0..6} (7 alike) : hdlBasic/Delay  rst=off  en=off  latency=1  reg_retiming=off  XmcBlockStatus=1  maskContainerNames=group1  block_type=delay  block_config=sysgen:Delay_config
  Enable Delay : hdlBasic/Delay  rst=off  en=off  latency=1  reg_retiming=off  XmcBlockStatus=1  maskContainerNames=group1  block_type=delay  block_config=sysgen:Delay_config
  FIFO 0 : hdlBasic/Constant  const=0  gui_display_data_type=Fixed-point  arith_type=Unsigned  n_bits=1  bin_pt=0  preci_type=Single  exp_width=8  frac_width=24  explicit_period=off  period=1  XmcBlockStatus=1  maskContainerNames=tabcontainer1  block_type=constant  block_config=sysgen:Constant_config
  FIFO 1 : hdlBasic/Constant  const=1  gui_display_data_type=Fixed-point  arith_type=Unsigned  n_bits=1  bin_pt=0  preci_type=Single  exp_width=8  frac_width=24  explicit_period=off  period=1  XmcBlockStatus=1  maskContainerNames=tabcontainer1  block_type=constant  block_config=sysgen:Constant_config
  FIFO 2 : hdlBasic/Constant  const=2  gui_display_data_type=Fixed-point  arith_type=Unsigned  n_bits=2  bin_pt=0  preci_type=Single  exp_width=8  frac_width=24  explicit_period=off  period=1  XmcBlockStatus=1  maskContainerNames=tabcontainer1  block_type=constant  block_config=sysgen:Constant_config
  Last Point Delay : hdlBasic/Delay  rst=off  en=off  latency=1  reg_retiming=off  XmcBlockStatus=1  maskContainerNames=group1  block_type=delay  block_config=sysgen:Delay_config
  Last Value Bypass FIFO 0 : hdlBasic/Logical  logical_function=OR  inputs=2  en=off  latency=1  precision=Full  arith_type=Unsigned  n_bits=16  bin_pt=0  align_bp=on  overflow=[]  quantization=[]  XmcBlockStatus=1  maskContainerNames=tabcontainer1  block_type=logical  block_config=sysgen:Logical_config
  Last Value Bypass FIFO 1 : hdlBasic/Logical  logical_function=OR  inputs=2  en=off  latency=1  precision=Full  arith_type=Unsigned  n_bits=16  bin_pt=0  align_bp=on  overflow=[]  quantization=[]  XmcBlockStatus=1  maskContainerNames=tabcontainer1  block_type=logical  block_config=sysgen:Logical_config
  Last Value Bypass FIFO 2 : hdlBasic/Logical  logical_function=OR  inputs=2  en=off  latency=1  precision=Full  arith_type=Unsigned  n_bits=16  bin_pt=0  align_bp=on  overflow=[]  quantization=[]  XmcBlockStatus=1  maskContainerNames=tabcontainer1  block_type=logical  block_config=sysgen:Logical_config
  Logical : hdlBasic/Logical  logical_function=NOR  inputs=3  en=off  latency=1  precision=Full  arith_type=Unsigned  n_bits=16  bin_pt=0  align_bp=on  overflow=[]  quantization=[]  XmcBlockStatus=1  maskContainerNames=tabcontainer1  block_type=logical  block_config=sysgen:Logical_config
  Store in FIFO 0 : hdlBasic/Relational  mode=a=b  op_type=Bool  en=off  latency=1  XmcBlockStatus=1  maskContainerNames=tabcontainer1  block_type=relational  block_config=sysgen:Relational_config
  Store in FIFO 1 : hdlBasic/Relational  mode=a=b  op_type=Bool  en=off  latency=1  XmcBlockStatus=1  maskContainerNames=tabcontainer1  block_type=relational  block_config=sysgen:Relational_config
  Store in FIFO 2 : hdlBasic/Relational  mode=a=b  op_type=Bool  en=off  latency=1  XmcBlockStatus=1  maskContainerNames=tabcontainer1  block_type=relational  block_config=sysgen:Relational_config
  Sync Frame Counter : hdlBasic/Counter  cnt_type=Count limited  cnt_to=2  operation=Up  start_count=0  cnt_by_val=1  arith_type=Unsigned  n_bits=2  bin_pt=0  load_pin=off  rst=on  en=on  explicit_period=Explicit  period=1  use_behavioral_HDL=off  implementation=Fabric  XmcBlockStatus=1  maskContainerNames=group1  block_type=counter  block_config=sysgen:Counter_config  block_width=531  block_height=1023
  Unpack Kernel 72 Bit FIFO 0 : Subsystem
      settings: RTWMemSecFuncInitTerm=Inherit fRAM model  RTWMemSecFuncExecute=Inherit fRAM model  RTWMemSecDataConstants=Inherit fRAM model  RTWMemSecDataInternal=Inherit fRAM model  RTWMemSecDataParameters=Inherit fRAM model
  Unpack Kernel 72 Bit FIFO 1 : Subsystem
      settings: RTWMemSecFuncInitTerm=Inherit fRAM model  RTWMemSecFuncExecute=Inherit fRAM model  RTWMemSecDataConstants=Inherit fRAM model  RTWMemSecDataInternal=Inherit fRAM model  RTWMemSecDataParameters=Inherit fRAM model
  Unpack Kernel 72 Bit FIFO 2 : Subsystem
      settings: RTWMemSecFuncInitTerm=Inherit fRAM model  RTWMemSecFuncExecute=Inherit fRAM model  RTWMemSecDataConstants=Inherit fRAM model  RTWMemSecDataInternal=Inherit fRAM model  RTWMemSecDataParameters=Inherit fRAM model
  Valid : hdlBasic/Delay  rst=off  en=off  latency=1  reg_retiming=off  XmcBlockStatus=1  maskContainerNames=group1  block_type=delay  block_config=sysgen:Delay_config
  Write to FIFO 0 : hdlBasic/Logical  logical_function=AND  inputs=2  en=off  latency=1  precision=Full  arith_type=Unsigned  n_bits=16  bin_pt=0  align_bp=on  overflow=[]  quantization=[]  XmcBlockStatus=1  maskContainerNames=tabcontainer1  block_type=logical  block_config=sysgen:Logical_config
  Write to FIFO 1 : hdlBasic/Logical  logical_function=AND  inputs=2  en=off  latency=1  precision=Full  arith_type=Unsigned  n_bits=16  bin_pt=0  align_bp=on  overflow=[]  quantization=[]  XmcBlockStatus=1  maskContainerNames=tabcontainer1  block_type=logical  block_config=sysgen:Logical_config
  Write to FIFO 2 : hdlBasic/Logical  logical_function=AND  inputs=2  en=off  latency=1  precision=Full  arith_type=Unsigned  n_bits=16  bin_pt=0  align_bp=on  overflow=[]  quantization=[]  XmcBlockStatus=1  maskContainerNames=tabcontainer1  block_type=logical  block_config=sysgen:Logical_config
  Zero Out : hdlBasic/Constant  const=0  gui_display_data_type=Fixed-point  arith_type=Unsigned  n_bits=72  bin_pt=0  preci_type=Single  exp_width=8  frac_width=24  explicit_period=off  period=1  XmcBlockStatus=1  maskContainerNames=tabcontainer1  block_type=constant  block_config=sysgen:Constant_config
  Zero Value : hdlBasic/Mux  inputs=2  en=off  latency=1  precision=Full  arith_type=Unsigned  n_bits=16  bin_pt=14  quantization=Truncate  overflow=Wrap  XmcBlockStatus=1  maskContainerNames=tabcontainer1  block_type=mux  block_config=sysgen:Mux_config
  71 Downto 54 FIFO 0 : Outport
  53 Downto 36 FIFO 0 : Outport  Port=2
  35 Downto 18 FIFO 0 : Outport  Port=3
  17 Downto 0 FIFO 0 : Outport  Port=4
  71 Downto 54 FIFO 1 : Outport  Port=5
  53 Downto 36 FIFO 1 : Outport  Port=6
  35 Downto 18 FIFO 1 : Outport  Port=7
  17 Downto 0 FIFO 1 : Outport  Port=8
  71 Downto 54 FIFO 2 : Outport  Port=9
  53 Downto 36 FIFO 2 : Outport  Port=10
  35 Downto 18 FIFO 2 : Outport  Port=11
  17 Downto 0 FIFO 2 : Outport  Port=12
  Valid Out : Outport  Port=13
  Wrote To a FIFO : Outport  Port=14
  wires:
  Sync Frame Counter/1 -> Store in FIFO 2/1, Store in FIFO 1/1, Store in FIFO 0/1
  Read Enable/1 -> 72bit Frame FIFO 0/3, 72bit Frame FIFO 1/3, 72bit Frame FIFO 2/3, Valid/1
  FIFO 1/1 -> Store in FIFO 1/2
  FIFO 0/1 -> Store in FIFO 0/2
  Data Delay 0/1 -> Data Delay 1/1
  Data In/1 -> Data Delay 0/1
  Enable/1 -> Enable Delay/1, Sync Frame Counter/2
  72bit Frame FIFO 0/1 -> Unpack Kernel 72 Bit FIFO 0/1(72 Bit Input)
  Unpack Kernel 72 Bit FIFO 0/1(71 Downto 54) -> 71 Downto 54 FIFO 0/1
  Unpack Kernel 72 Bit FIFO 0/2(53 Downto 36) -> 53 Downto 36 FIFO 0/1
  Unpack Kernel 72 Bit FIFO 0/3(35 Downto 18) -> 35 Downto 18 FIFO 0/1
  Unpack Kernel 72 Bit FIFO 0/4(17 Downto 0) -> 17 Downto 0 FIFO 0/1
  Valid/1 -> Valid Out/1
  FIFO 2/1 -> Store in FIFO 2/2
  Unpack Kernel 72 Bit FIFO 1/3(35 Downto 18) -> 35 Downto 18 FIFO 1/1
  Unpack Kernel 72 Bit FIFO 1/2(53 Downto 36) -> 53 Downto 36 FIFO 1/1
  Unpack Kernel 72 Bit FIFO 1/1(71 Downto 54) -> 71 Downto 54 FIFO 1/1
  Unpack Kernel 72 Bit FIFO 1/4(17 Downto 0) -> 17 Downto 0 FIFO 1/1
  72bit Frame FIFO 1/1 -> Unpack Kernel 72 Bit FIFO 1/1(72 Bit Input)
  Unpack Kernel 72 Bit FIFO 2/3(35 Downto 18) -> 35 Downto 18 FIFO 2/1
  Unpack Kernel 72 Bit FIFO 2/2(53 Downto 36) -> 53 Downto 36 FIFO 2/1
  Unpack Kernel 72 Bit FIFO 2/1(71 Downto 54) -> 71 Downto 54 FIFO 2/1
  Unpack Kernel 72 Bit FIFO 2/4(17 Downto 0) -> 17 Downto 0 FIFO 2/1
  72bit Frame FIFO 2/1 -> Unpack Kernel 72 Bit FIFO 2/1(72 Bit Input)
  Last Value Bypass FIFO 0/1 -> Write to FIFO 0/1
  Last Value Bypass FIFO 1/1 -> Write to FIFO 1/2
  Bypass Delay/1 -> Write to FIFO 1/1, Write to FIFO 2/1, Write to FIFO 0/2
  Last Value Bypass FIFO 2/1 -> Write to FIFO 2/2
  Write to FIFO 0/1 -> Data Delay 4/1
  Write to FIFO 1/1 -> Data Delay 5/1
  Write to FIFO 2/1 -> Data Delay 6/1
  Store in FIFO 0/1 -> Last Value Bypass FIFO 0/2
  Store in FIFO 1/1 -> Last Value Bypass FIFO 1/1
  Store in FIFO 2/1 -> Last Value Bypass FIFO 2/1
  Enable Delay/1 -> Bypass Delay/1
  Last Point/1 -> Last Point Delay/1, Sync Frame Counter/1
  Last Point Delay/1 -> Last Value Bypass FIFO 2/2, Last Value Bypass FIFO 0/1, Bypass Delay1/1, Last Value Bypass FIFO 1/2
  Data Delay 1/1 -> Data Delay 2/1
  Data Delay 2/1 -> Data Delay 3/1, Zero Value/2
  Logical/1 -> Wrote To a FIFO/1
  72bit Frame FIFO 1/2 -> Logical/1
  72bit Frame FIFO 2/2 -> Logical/2
  72bit Frame FIFO 0/2 -> Logical/3
  Zero Value/1 -> 72bit Frame FIFO 1/1, 72bit Frame FIFO 2/1
  Data Delay 3/1 -> 72bit Frame FIFO 0/1
  Data Delay 4/1 -> 72bit Frame FIFO 0/2
  Data Delay 5/1 -> 72bit Frame FIFO 1/2
  Data Delay 6/1 -> 72bit Frame FIFO 2/2
  Zero Out/1 -> Zero Value/3
  Bypass Delay1/1 -> Bypass Delay2/1
  Bypass Delay2/1 -> Zero Value/1
